simulink model "sim3"  (R2020b)
settings: Solver=VariableStepAuto  StartTime=0.0  StopTime=50  RelTol=1e-3
undefined symbols (not defined in the file): h, ym
settings Model: Creator=48576  LastModifiedBy=48576

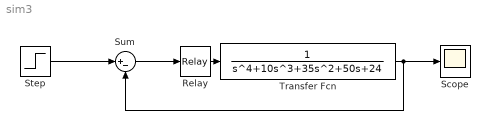
== system sim3 ==
  Relay : Relay  OnSwitchValue=h  OffSwitchValue=-h  OnOutputValue=ym  OffOutputValue=-ym
  Scope : Scope
  Step : Step  SampleTime=0
  Sum : Sum  Inputs=|+-
  Transfer Fcn : TransferFcn  Denominator=[1 10 35 50 24]
  wires:
  Step/1 -> Sum/1
  Sum/1 -> Relay/1
  Relay/1 -> Transfer Fcn/1
  Transfer Fcn/1 -> Scope/1, Sum/2
